simulink model "RmtAPP_Plaus12"  (R2016b)
settings: configuration reference "CodeGenConfigSet" (kept outside this file)
values from neighbouring files (symbols this model uses):
  MoFRmtAPP_dRawSigFac_C = Calibration.Parameter    [init_RmtAPP_Plaus12.m]    (also in init_RmtAPP_Plaus12_SIL.m = Simulink.Parameter)
  MoFRmtAPP_uSync_CUR = Calibration.Parameter    [init_RmtAPP_Plaus12.m]    (also in init_RmtAPP_Plaus12_SIL.m = Simulink.Parameter)
  MoFRmtAPP_uSync_CURX = Calibration.Parameter    [init_RmtAPP_Plaus12.m]    (also in init_RmtAPP_Plaus12_SIL.m = Simulink.Parameter)
  RmtAPP_PlaAPPDefDeb_C = Calibration.Parameter    [init_RmtAPP_Plaus12.m]    (also in init_RmtAPP_Plaus12_SIL.m = Simulink.Parameter)
  RmtAPP_PlaAPPDefOK_C = Calibration.Parameter    [init_RmtAPP_Plaus12.m]    (also in init_RmtAPP_Plaus12_SIL.m = Simulink.Parameter)
  RmtAPP_uSyncMin_C = Calibration.Parameter    [init_RmtAPP_Plaus12.m]    (also in init_RmtAPP_Plaus12_SIL.m = Simulink.Parameter)
undefined symbols (not defined in the file or in its folder): RmtAPP_Plaus12_DT
libraries: CXLib x3
settings Model: Creator=bianxuyin  LastModifiedBy=bianxuyin
settings ConfigSetRef: SourceLocation=Base Workspace

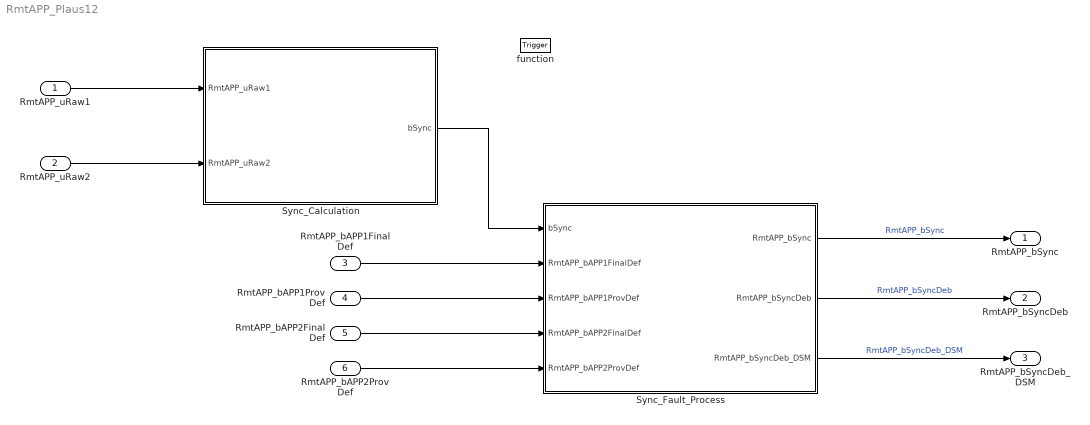
== system RmtAPP_Plaus12 ==
  RmtAPP_uRaw1 : Inport  Tag=mv  Description=Remote Acceleration Pedal Position D  OutMin=0  OutMax=5000  OutDataTypeStr=Ad_mv
  RmtAPP_uRaw2 : Inport  Tag=mv  Description=Remote Acceleration Pedal Position E  Port=2  OutMin=0  OutMax=5000  OutDataTypeStr=Ad_mv
  RmtAPP_bAPP1FinalDef : Inport  Description=Status Sensor 1 of the remote acceleration pedal finally defect  Port=3  OutMin=0  OutMax=1  OutDataTypeStr=boolean
  RmtAPP_bAPP1ProvDef : Inport  Description=Status Sensor 1 of the remot acceleration pedal temporary defect  Port=4  OutMin=0  OutMax=1  OutDataTypeStr=boolean
  RmtAPP_bAPP2FinalDef : Inport  Description=Status Sensor 2 of the remote acceleration pedal finally defect  Port=5  OutMin=0  OutMax=1  OutDataTypeStr=boolean
  RmtAPP_bAPP2ProvDef : Inport  Description=Status Sensor 2 of the remote acceleration pedal temporary defect  Port=6  OutMin=0  OutMax=1  OutDataTypeStr=boolean
  function : TriggerPort  TriggerType=function-call  VariantControl=Variant
  Sync_Calculation : Subsystem
  Sync_Fault_Process : Subsystem
  RmtAPP_bSync : Outport  Description=Status temporary sync check  OutMin=0  OutMax=1  OutDataTypeStr=boolean
  RmtAPP_bSyncDeb : Outport  Description=Status debounced sync check  Port=2  OutMin=0  OutMax=1  OutDataTypeStr=boolean
  RmtAPP_bSyncDeb_DSM : Outport  Description=Status debounced sync check finally defect  Port=3  OutMin=0  OutMax=1  OutDataTypeStr=boolean
  wires:
  Sync_Fault_Process/1(RmtAPP_bSync) -> RmtAPP_bSync/1  "RmtAPP_bSync"
  Sync_Fault_Process/2(RmtAPP_bSyncDeb) -> RmtAPP_bSyncDeb/1  "RmtAPP_bSyncDeb"
  Sync_Fault_Process/3(RmtAPP_bSyncDeb_DSM) -> RmtAPP_bSyncDeb_DSM/1  "RmtAPP_bSyncDeb_DSM"
  RmtAPP_uRaw1/1 -> Sync_Calculation/1(RmtAPP_uRaw1)
  RmtAPP_uRaw2/1 -> Sync_Calculation/2(RmtAPP_uRaw2)
  Sync_Calculation/1(bSync) -> Sync_Fault_Process/1(bSync)
  RmtAPP_bAPP1FinalDef/1 -> Sync_Fault_Process/2(RmtAPP_bAPP1FinalDef)
  RmtAPP_bAPP1ProvDef/1 -> Sync_Fault_Process/3(RmtAPP_bAPP1ProvDef)
  RmtAPP_bAPP2FinalDef/1 -> Sync_Fault_Process/4(RmtAPP_bAPP2FinalDef)
  RmtAPP_bAPP2ProvDef/1 -> Sync_Fault_Process/5(RmtAPP_bAPP2ProvDef)

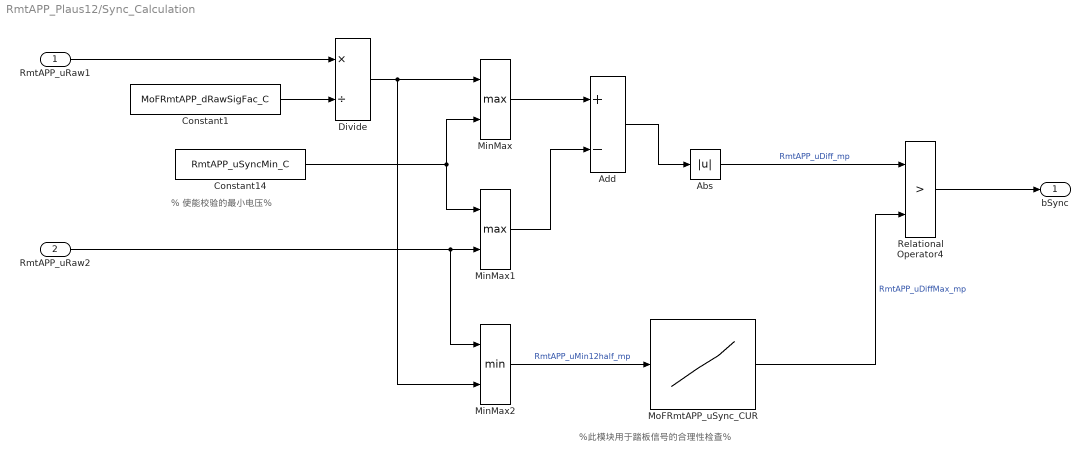
== system RmtAPP_Plaus12/Sync_Calculation ==
  note: %此模块用于踏板信号的合理性检查%
  note: % 使能校验的最小电压%
  RmtAPP_uRaw1 : Inport
  RmtAPP_uRaw2 : Inport  Port=2
  Abs : Abs  OutDataTypeStr=Inherit: Inherit via back propagation
  Add : Sum  Inputs=+-  InputSameDT=on
  Constant1 : Constant  Value=MoFRmtAPP_dRawSigFac_C  SampleTime=-1
  Constant14 : Constant  Value=RmtAPP_uSyncMin_C  SampleTime=-1
  Divide : Product  Inputs=*/  OutDataTypeStr=Ad_mv
  MinMax : MinMax  Function=max  Inputs=2  InputSameDT=on
  MinMax1 : MinMax  Function=max  Inputs=2  InputSameDT=on
  MinMax2 : MinMax  Inputs=2  InputSameDT=on
  MoFRmtAPP_uSync_CUR : Lookup_n-D  NumberOfTableDimensions=1  BreakpointsForDimension1=MoFRmtAPP_uSync_CURX  IndexSearchMethod=Linear search  BeginIndexSearchUsingPreviousIndexResult=on  Table=MoFRmtAPP_uSync_CUR  ExtrapMethod=Clip  UseLastTableValue=on  InternalRulePriority=Speed  OutDataTypeStr=Inherit: Inherit via back propagation  SaturateOnIntegerOverflow=on  MaximumIndicesForEachDimension=MoFAPP_uSync_CURMAX
  Relational Operator4 : RelationalOperator  Operator=>  OutDataTypeStr=boolean  RndMeth=Nearest  InputSameDT=on
  bSync : Outport
  wires:
  Relational Operator4/1 -> bSync/1
  MinMax2/1 -> MoFRmtAPP_uSync_CUR/1  "RmtAPP_uMin12half_mp"
  MinMax1/1 -> Add/2
  Divide/1 -> MinMax/1, MinMax2/2
  MinMax/1 -> Add/1
  RmtAPP_uRaw2/1 -> MinMax2/1, MinMax1/2
  Abs/1 -> Relational Operator4/1  "RmtAPP_uDiff_mp"
  Constant14/1 -> MinMax/2, MinMax1/1
  RmtAPP_uRaw1/1 -> Divide/1
  MoFRmtAPP_uSync_CUR/1 -> Relational Operator4/2  "RmtAPP_uDiffMax_mp"
  Constant1/1 -> Divide/2
  Add/1 -> Abs/1

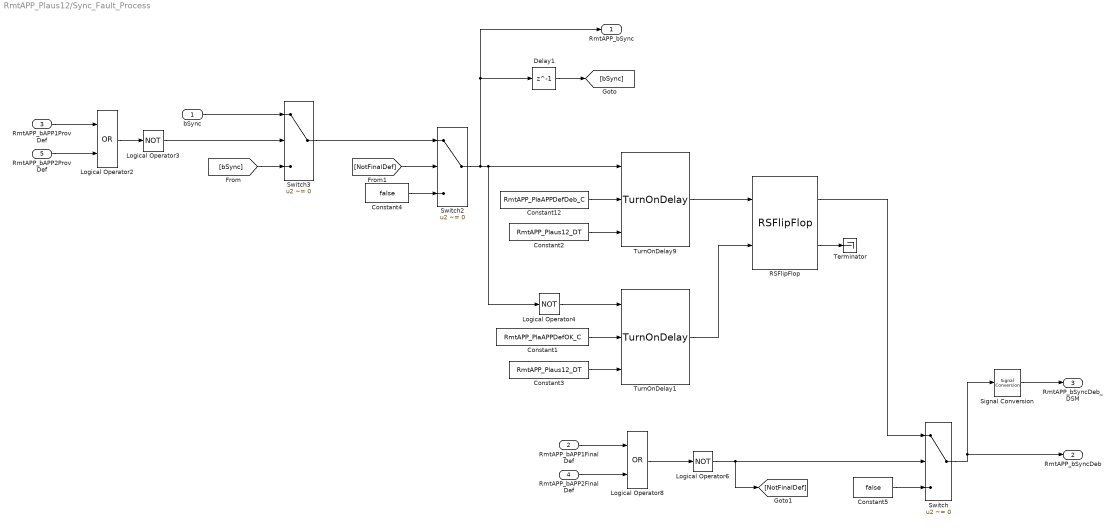
== system RmtAPP_Plaus12/Sync_Fault_Process ==
  bSync : Inport
  RmtAPP_bAPP1FinalDef : Inport  Tag=-  Description=Status Sensor 1 of the acceleration pedal finally defect  Port=2  OutMin=0  OutMax=1  OutDataTypeStr=boolean
  RmtAPP_bAPP1ProvDef : Inport  Tag=-  Description=Status Sensor 1 of the acceleration pedal temporary defect  Port=3  OutMin=0  OutMax=1  OutDataTypeStr=boolean
  RmtAPP_bAPP2FinalDef : Inport  Tag=-  Description=Status Sensor 2 of the acceleration pedal finally defect  Port=4  OutMin=0  OutMax=1  OutDataTypeStr=boolean
  RmtAPP_bAPP2ProvDef : Inport  Tag=-  Description=Status Sensor 2 of the acceleration pedal temporary defect  Port=5  OutMin=0  OutMax=1  OutDataTypeStr=boolean
  Constant1 : Constant  Value=RmtAPP_PlaAPPDefOK_C
  Constant12 : Constant  Value=RmtAPP_PlaAPPDefDeb_C
  Constant2 : Constant  Value=RmtAPP_Plaus12_DT  OutDataTypeStr=Inherit: Inherit via back propagation
  Constant3 : Constant  Value=RmtAPP_Plaus12_DT  OutDataTypeStr=Inherit: Inherit via back propagation
  Constant4 : Constant  Value=false  OutDataTypeStr=boolean
  Constant5 : Constant  Value=false  OutDataTypeStr=boolean
  Delay1 : Delay  DelayLength=1  InitialCondition=0  StateName=time
  Logical Operator2 : Logic  Operator=OR  OutDataTypeStr=boolean
  Logical Operator3 : Logic  Operator=NOT  AllPortsSameDT=off  OutDataTypeStr=boolean
  Logical Operator4 : Logic  Operator=NOT  AllPortsSameDT=off  OutDataTypeStr=boolean
  Logical Operator6 : Logic  Operator=NOT  AllPortsSameDT=off  OutDataTypeStr=boolean
  Logical Operator8 : Logic  Operator=OR  OutDataTypeStr=boolean
  RSFlipFlop : CXLib/RSFlipFlop
  Signal Conversion : SignalConversion  OverrideOpt=off
  Switch : Switch  Criteria=u2 ~= 0  InputSameDT=on
  Switch2 : Switch  Criteria=u2 ~= 0  InputSameDT=on
  Switch3 : Switch  Criteria=u2 ~= 0  InputSameDT=on
  Terminator : Terminator
  TurnOnDelay1 : CXLib/TurnOnDelay
  TurnOnDelay9 : CXLib/TurnOnDelay
  RmtAPP_bSync : Outport  Tag=-  Description=Status temporary sync check  OutMin=0  OutMax=1  OutDataTypeStr=boolean
  RmtAPP_bSyncDeb : Outport  Tag=-  Description=Status debounced sync check  Port=2  OutMin=0  OutMax=1  OutDataTypeStr=boolean
  RmtAPP_bSyncDeb_DSM : Outport  Tag=-  Description=Status debounced sync check  Port=3  OutMin=0  OutMax=1  OutDataTypeStr=boolean
  wires:
  bSync/1 -> Switch3/1
  Delay1/1 -> [bSync]
  RSFlipFlop/1 -> Switch/1
  Logical Operator2/1 -> Logical Operator3/1
  Constant5/1 -> Switch/3
  Logical Operator8/1 -> Logical Operator6/1
  RmtAPP_bAPP2ProvDef/1 -> Logical Operator2/2
  RmtAPP_bAPP2FinalDef/1 -> Logical Operator8/2
  RmtAPP_bAPP1FinalDef/1 -> Logical Operator8/1
  Logical Operator6/1 -> [NotFinalDef], Switch/2
  RmtAPP_bAPP1ProvDef/1 -> Logical Operator2/1
  [NotFinalDef] -> Switch2/2
  Switch3/1 -> Switch2/1
  Constant4/1 -> Switch2/3
  Switch/1 -> RmtAPP_bSyncDeb/1, Signal Conversion/1
  Logical Operator3/1 -> Switch3/2
  Signal Conversion/1 -> RmtAPP_bSyncDeb_DSM/1
  Constant3/1 -> TurnOnDelay1/3
  Constant2/1 -> TurnOnDelay9/3
  RSFlipFlop/2 -> Terminator/1
  Switch2/1 -> TurnOnDelay9/1, Logical Operator4/1, Delay1/1, RmtAPP_bSync/1
  Logical Operator4/1 -> TurnOnDelay1/1
  TurnOnDelay1/1 -> RSFlipFlop/2
  Constant1/1 -> TurnOnDelay1/2
  Constant12/1 -> TurnOnDelay9/2
  TurnOnDelay9/1 -> RSFlipFlop/1
  [bSync] -> Switch3/3
